simulink model "simulation"  (R2015a)
settings: Solver=ode45  StartTime=0.0  StopTime=20  RelTol=1e-3
values from neighbouring files (symbols this model uses):
  a = g/l    (= 32.1639344262)    [constants.m]    (also in lyapRedesign.m = -32.1639344262; smc.m = -32.1639344262)
  b = kf/m    (= 5)    [constants.m]
  c = 1/(l^2*m)    (= 107.497984413)    [constants.m]
  epsilon = 0.1    [constants.m]
  kappa = 0.05    [constants.m]
libraries: simulink x1
settings Model: Creator=Nikolaj  LastModifiedBy=Nikolaj

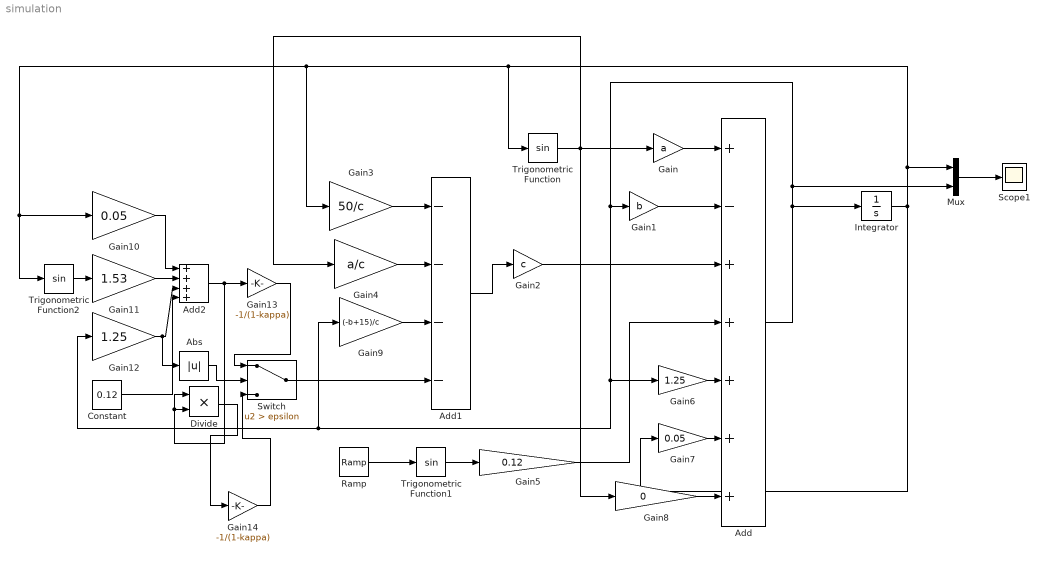
== system simulation ==
  Abs : Abs
  Add : Sum  Inputs=+-+++++
  Add1 : Sum  Inputs=----
  Add2 : Sum  Inputs=++++
  Constant : Constant  Value=0.12
  Divide : Product  Inputs=**
  Gain : Gain  Gain=a
  Gain1 : Gain  Gain=b
  Gain10 : Gain  Gain=0.05
  Gain11 : Gain  Gain=1.53
  Gain12 : Gain  Gain=1.25
  Gain13 : Gain  Gain=-1/(1-kappa)
  Gain14 : Gain  Gain=-1/(1-kappa)
  Gain2 : Gain  Gain=c
  Gain3 : Gain  Gain=50/c
  Gain4 : Gain  Gain=a/c
  Gain5 : Gain  Gain=0.12
  Gain6 : Gain  Gain=1.25
  Gain7 : Gain  Gain=0.05
  Gain8 : Gain  Gain=0
  Gain9 : Gain  Gain=(-b+15)/c
  Integrator : Integrator  InitialCondition=pi/4
  Mux : Mux  Inputs=2
  Ramp : simulink/Sources/Ramp  slope=1  start=0  X0=0
  Scope1 : Scope
      settings: YMin=-16  YMax=2
  Switch : Switch  Criteria=u2 > Threshold  Threshold=epsilon  ZeroCross=off
  Trigonometric Function : Trigonometry
  Trigonometric Function1 : Trigonometry
  Trigonometric Function2 : Trigonometry
  wires:
  Add/1 -> Gain12/1, Gain9/1, Gain6/1, Gain1/1, Mux/2, Integrator/1
  Trigonometric Function/1 -> Gain8/1, Gain4/1, Gain/1
  Gain/1 -> Add/1
  Gain1/1 -> Add/2
  Gain2/1 -> Add/3
  Add1/1 -> Gain2/1
  Gain3/1 -> Add1/1
  Gain4/1 -> Add1/2
  Mux/1 -> Scope1/1
  Integrator/1 -> Mux/1, Trigonometric Function/1, Gain3/1, Trigonometric Function2/1, Gain10/1, Gain7/1
  Ramp/1 -> Trigonometric Function1/1
  Trigonometric Function1/1 -> Gain5/1
  Gain5/1 -> Add/4
  Gain6/1 -> Add/5
  Gain7/1 -> Add/6
  Gain8/1 -> Add/7
  Gain9/1 -> Add1/3
  Switch/1 -> Add1/4
  Gain10/1 -> Add2/1
  Gain11/1 -> Add2/2
  Trigonometric Function2/1 -> Gain11/1
  Constant/1 -> Add2/4
  Gain12/1 -> Abs/1, Add2/3
  Gain13/1 -> Switch/1
  Add2/1 -> Divide/2, Divide/1, Gain13/1
  Divide/1 -> Gain14/1
  Gain14/1 -> Switch/3
  Abs/1 -> Switch/2
